simulink model "EffectuatorIntegratedWithDemonstrator"  (R2020a)
settings: Solver=FixedStepDiscrete  StartTime=0.0  StopTime=inf  FixedStep=Ts  RelTol=1e-3
InitFcn:
  | %% Verwende vordefinierte Setpoints (Kreis mit Z-Komponente)
  | 
  | % Config
  | numCircles = 3;
  | scale=6;
  | %Versuch symmetrische Setpunkte zu setzen
  | pointsPerCircle =scale*(4+3*numCircles)+2;
  | 
  | r = 50;
  | m_x = r;
  | m_y = r;
  | 
  | % //
  | s = linspace(0,2*pi,pointsPerCircle);
  | 
  | setPoints_x = [];
  | setPoints_y = [];
  | 
  | for ii=1:numCircles
  | 
  | setPoints_x = [setPoints_x (-cos(s(1:floor(pointsPerCircle / 2))).*r + m_x + 2*r*(ii-1))]; %#ok<AGROW>
  | setPoints_y = [setPoints_y (sin(s).*r+m_y)]; %#ok<AGROW>pointsPerCircle / 2
  | 
  | end
  | 
  | setPoints_x = [setPoints_x flip(setPoints_x(1:end))];
  | 
  | % Loeschen doppelter y-Werte (Kreisuebergang)
  | setPoints_x(pointsPerCircle .* [1:numCircles]) = [];
  | setPoints_y(pointsPerCircle .* [1:numCircles]) = [];
  | 
  | % setPoints_x= [linspace(0,setPoints_x(19),19) setPoints_x(20:end)];
  | % setPoints_y= [linspace(0,setPoints_y(19),19) setPoints_y(20:end)];
  | 
  | % Array Elemente verschieben
  | % setPoints_x = circshift(setPoints_x,-pointsPerCircle/4,2);
  | % setPoints_y = circshift(setPoints_y,-pointsPerCircle/4,2);
  | 
  | z = zeros(1,size(setPoints_x,2));
  | z_x = -5:5;
  | z_y = -z_x.^2 + 25;
  | z_idx = 90;
  | z_idx2 = 210;
  | z(z_idx:z_idx+length(z_x)-1) = z_y;
  | z(z_idx2:z_idx2+length(z_x)-1) = z_y;
  | % z = [z_y z];
  | setPoints_z = z;
  | 
  | % setPoints_x = [zeros(1,length(z_y)) setPoints_x];
  | % setPoints_y = [setPoints_y(1,1)*ones(1,length(z_y)) setPoints_y];
  | 
  | % Umrechnung der Einheiten für Demonstrator
  | % setPoints_x = setPoints_x ./ 1000;
  | % setPoints_y = setPoints_y ./ 1000;
  | % setPoints_z = setPoints_z ./ 1000;
  | 
  | 
  | %{
  | plot(setPoints_x,setPoints_y);
  | fig = figure;
  | ... (+13 lines)
StartFcn:
  | close all;
model workspace (MAT data in the model file):
  MvmtPerfEval_collectVal : Simulink.Parameter (value not decoded)
  MvmtPerfEval_sendOwnVal : Simulink.Parameter (value not decoded)
  PerfEval_numTicks_enable : Simulink.Parameter (value not decoded)
  Segmentregler_I_Gain : Simulink.Parameter (value not decoded)
  Segmentregler_P_Gain : Simulink.Parameter (value not decoded)
  Segmentregler_minVel_enable : Simulink.Parameter (value not decoded)
  Segmentregler_numTicks_enable : Simulink.Parameter (value not decoded)
  Ts : Simulink.Parameter (value not decoded)
  maxPos_x : Simulink.Parameter (value not decoded)
  maxPos_y : Simulink.Parameter (value not decoded)
  maxPos_z : Simulink.Parameter (value not decoded)
  maxVectorLengths : Simulink.Parameter (value not decoded)
  minAllowedVelSaturation : Simulink.Parameter (value not decoded)
  numAxes : Simulink.Parameter (value not decoded)
symbols that are objects in the model workspace (value not decoded): maxPos_x, maxPos_y, maxPos_z, minAllowedVelSaturation, MvmtPerfEval_collectVal, MvmtPerfEval_sendOwnVal, numAxes, PerfEval_numTicks_enable, Segmentregler_I_Gain, Segmentregler_minVel_enable, Segmentregler_numTicks_enable, Segmentregler_P_Gain, Ts
undefined symbols (not defined in the file or in its folder): DiscIntNeverNeededParam, VelOverride
libraries: simulink x20, vrlib x5, sldrtlib x2, xpcrtudplib x2, dspnetwork x2, ptplib x1, etargetslib x1, xpcutilitieslib x1
(part 2 of 5)

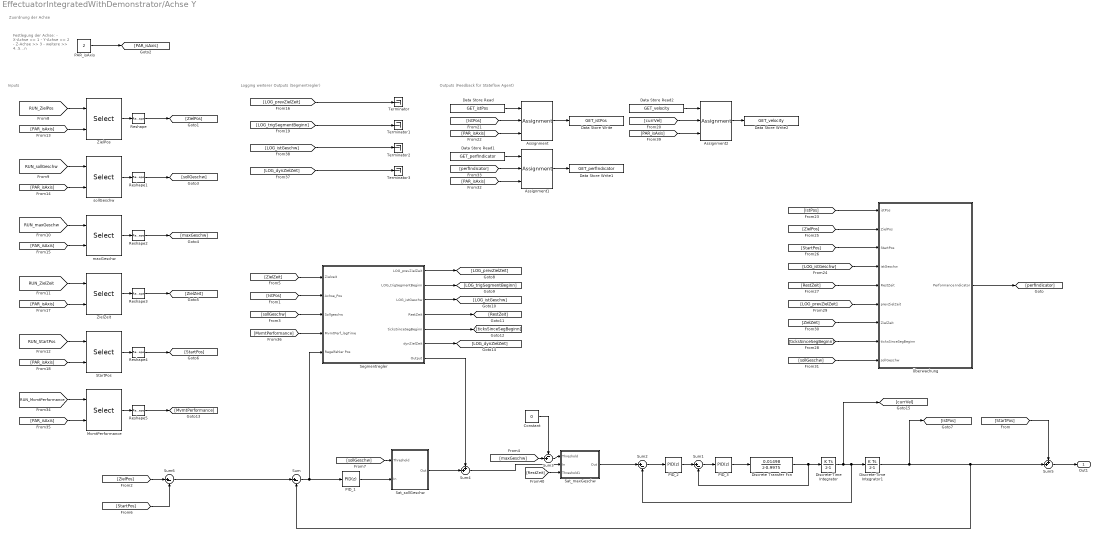
== system EffectuatorIntegratedWithDemonstrator/Achse Y ==
  note: Inputs
  note: Festlegung der Achse:
      | - X-Achse >> 1
      | - Y-Achse >> 2
      | - Z-Achse >> 3
      | - weitere >> 4..5...n
  note: Zuordnung der Achse
  note: Logging weiterer Outputs (Segmentregler)
  note: Outputs (Feedback für Stateflow Agent)
  Assignment : Assignment  DiagnosticForDimensions=Warning  IndexOptions=Index vector (port)  Indices=1  OutputSizes=1
  Assignment1 : Assignment  DiagnosticForDimensions=Warning  IndexOptions=Index vector (port)  Indices=1  OutputSizes=1
  Assignment2 : Assignment  DiagnosticForDimensions=Warning  IndexOptions=Index vector (port)  Indices=1  OutputSizes=1
  Constant : Constant  Value=0
  Data Store Read : DataStoreRead  DataStoreName=GET_istPos
  Data Store Read1 : DataStoreRead  DataStoreName=GET_perfIndicator
  Data Store Read2 : DataStoreRead  DataStoreName=GET_velocity
  Data Store Write : DataStoreWrite  DataStoreName=GET_istPos
  Data Store Write1 : DataStoreWrite  DataStoreName=GET_perfIndicator
  Data Store Write2 : DataStoreWrite  DataStoreName=GET_velocity
  Discrete Transfer Fcn : DiscreteTransferFcn  Numerator=0.01498  Denominator=[1 -0.9975]
  Discrete-Time Integrator : DiscreteIntegrator  SampleTime=-1  ICPrevOutput=DiscIntNeverNeededParam  ICPrevScaledInput=DiscIntNeverNeededParam
  Discrete-Time Integrator1 : DiscreteIntegrator  SampleTime=-1  ICPrevOutput=DiscIntNeverNeededParam  ICPrevScaledInput=DiscIntNeverNeededParam
  MvmtPerformance : Selector  IndexOptions=Index vector (port)  Indices=[1 3]  OutputSizes=1
  PAR_isAxis : Constant  Value=2
  PID_1 : simulink/Continuous/PID Controller  Controller=PID  Form=Parallel  TimeDomain=Discrete-time  UseExternalTs=off  SampleTime=-1  IntegratorMethod=Forward Euler  FilterMethod=Forward Euler  ControllerParametersSource=internal  P=20  I=0  D=0  UseFilter=on  N=100  TunerSelectOption=Transfer Function Based (PID Tuner App)  InitialConditionSource=internal  InitialConditionForIntegrator=0  InitialConditionForFilter=0  DifferentiatorICPrevScaledInput=0  ExternalReset=none  TrackingMode=off  Kt=1  LimitOutput=off  UpperSaturationLimit=inf  LowerSaturationLimit=-inf  LinearizeAsGain=off  AntiWindupMode=none  Kb=1  POutMin=[]  POutMax=[]  IOutMin=[]  IOutMax=[]  DOutMin=[]  DOutMax=[]  NOutMin=[]  NOutMax=[]  SumOutMin=[]  SumOutMax=[]  SaturationOutMin=[]  SaturationOutMax=[]  PParamMin=[]  PParamMax=[]  IParamMin=[]  IParamMax=[]  DParamMin=[]  DParamMax=[]  NParamMin=[]  NParamMax=[]  KbParamMin=[]  KbParamMax=[]  KtParamMin=[]  KtParamMax=[]  KbOutMin=[]  KbOutMax=[]  KtOutMin=[]  KtOutMax=[]  IntegratorOutMin=[]  IntegratorOutMax=[]  FilterOutMin=[]  FilterOutMax=[]  SumI1OutMin=[]  SumI1OutMax=[]  SumI2OutMin=[]  SumI2OutMax=[]  SumI3OutMin=[]  SumI3OutMax=[]  SumI4OutMin=[]  SumI4OutMax=[]  SumDOutMin=[]  SumDOutMax=[]  DifferentiatorOutMin=[]  DifferentiatorOutMax=[]  FilterDiffOutCoefMin=[]  FilterDiffOutCoefMax=[]  ReciprocalOutMin=[]  ReciprocalOutMax=[]  SumDenOutMin=[]  SumDenOutMax=[]  SumNumOutMin=[]  SumNumOutMax=[]  DivideOutMin=[]  DivideOutMax=[]  UdiffTsProdOutMin=[]  UdiffTsProdOutMax=[]  NTsProdOutMin=[]  NTsProdOutMax=[]  UintegralTsProdOutMin=[]  UintegralTsProdOutMax=[]  UngainTsProdOutMin=[]  UngainTsProdOutMax=[]  IntegratorContinuousStateAttributes=''  IntegratorStateMustResolveToSignalObject=off  IntegratorRTWStateStorageClass=Auto  FilterContinuousStateAttributes=''  FilterStateMustResolveToSignalObject=off  FilterRTWStateStorageClass=Auto  ParallelPVariant=InternalParameters  IdealPVariant=Disabled  IVariant=InternalParameters  DVariant=InternalParameters  IntegratorVariant=Discrete  SatVariant=Disabled  AWVariant=Passthrough  PCopyVariant=Disabled  TRVariant=Disabled  FdbkBlocksVariant=Forward  IdealPFdbkVariant=Disabled  SatFdbkVariant=Disabled  DerivativeFilterVariant=ForwardEulerFilter  NVariant=InternalParameters  NCopyVariant=Disabled  FilterICVariant=InternalICsFilter  IntegratorICVariant=InternalICs  ExternalResetVariant=Disabled  TRSumVariant=Passthrough  SumFdbkVariant=Disabled  SumVariant=Sum_PID  TsampFilterVariant=InternalTs  TsampNgainVariant=Passthrough  TsampIntegralVariant=Passthrough
  PID_2 : simulink/Continuous/PID Controller  Controller=PID  Form=Parallel  TimeDomain=Discrete-time  UseExternalTs=off  SampleTime=-1  IntegratorMethod=Forward Euler  FilterMethod=Forward Euler  ControllerParametersSource=internal  P=20  I=1  D=0  UseFilter=on  N=100  TunerSelectOption=Transfer Function Based (PID Tuner App)  InitialConditionSource=internal  InitialConditionForIntegrator=0  InitialConditionForFilter=0  DifferentiatorICPrevScaledInput=0  ExternalReset=none  TrackingMode=off  Kt=1  LimitOutput=off  UpperSaturationLimit=inf  LowerSaturationLimit=-inf  LinearizeAsGain=off  AntiWindupMode=none  Kb=1  POutMin=[]  POutMax=[]  IOutMin=[]  IOutMax=[]  DOutMin=[]  DOutMax=[]  NOutMin=[]  NOutMax=[]  SumOutMin=[]  SumOutMax=[]  SaturationOutMin=[]  SaturationOutMax=[]  PParamMin=[]  PParamMax=[]  IParamMin=[]  IParamMax=[]  DParamMin=[]  DParamMax=[]  NParamMin=[]  NParamMax=[]  KbParamMin=[]  KbParamMax=[]  KtParamMin=[]  KtParamMax=[]  KbOutMin=[]  KbOutMax=[]  KtOutMin=[]  KtOutMax=[]  IntegratorOutMin=[]  IntegratorOutMax=[]  FilterOutMin=[]  FilterOutMax=[]  SumI1OutMin=[]  SumI1OutMax=[]  SumI2OutMin=[]  SumI2OutMax=[]  SumI3OutMin=[]  SumI3OutMax=[]  SumI4OutMin=[]  SumI4OutMax=[]  SumDOutMin=[]  SumDOutMax=[]  DifferentiatorOutMin=[]  DifferentiatorOutMax=[]  FilterDiffOutCoefMin=[]  FilterDiffOutCoefMax=[]  ReciprocalOutMin=[]  ReciprocalOutMax=[]  SumDenOutMin=[]  SumDenOutMax=[]  SumNumOutMin=[]  SumNumOutMax=[]  DivideOutMin=[]  DivideOutMax=[]  UdiffTsProdOutMin=[]  UdiffTsProdOutMax=[]  NTsProdOutMin=[]  NTsProdOutMax=[]  UintegralTsProdOutMin=[]  UintegralTsProdOutMax=[]  UngainTsProdOutMin=[]  UngainTsProdOutMax=[]  IntegratorContinuousStateAttributes=''  IntegratorStateMustResolveToSignalObject=off  IntegratorRTWStateStorageClass=Auto  FilterContinuousStateAttributes=''  FilterStateMustResolveToSignalObject=off  FilterRTWStateStorageClass=Auto  ParallelPVariant=InternalParameters  IdealPVariant=Disabled  IVariant=InternalParameters  DVariant=InternalParameters  IntegratorVariant=Discrete  SatVariant=Disabled  AWVariant=Passthrough  PCopyVariant=Disabled  TRVariant=Disabled  FdbkBlocksVariant=Forward  IdealPFdbkVariant=Disabled  SatFdbkVariant=Disabled  DerivativeFilterVariant=ForwardEulerFilter  NVariant=InternalParameters  NCopyVariant=Disabled  FilterICVariant=InternalICsFilter  IntegratorICVariant=InternalICs  ExternalResetVariant=Disabled  TRSumVariant=Passthrough  SumFdbkVariant=Disabled  SumVariant=Sum_PID  TsampFilterVariant=InternalTs  TsampNgainVariant=Passthrough  TsampIntegralVariant=Passthrough
  PID_3 : simulink/Continuous/PID Controller  Controller=PID  Form=Parallel  TimeDomain=Discrete-time  UseExternalTs=off  SampleTime=-1  IntegratorMethod=Forward Euler  FilterMethod=Forward Euler  ControllerParametersSource=internal  P=20  I=1  D=0  UseFilter=on  N=100  TunerSelectOption=Transfer Function Based (PID Tuner App)  InitialConditionSource=internal  InitialConditionForIntegrator=0  InitialConditionForFilter=0  DifferentiatorICPrevScaledInput=0  ExternalReset=none  TrackingMode=off  Kt=1  LimitOutput=off  UpperSaturationLimit=inf  LowerSaturationLimit=-inf  LinearizeAsGain=off  AntiWindupMode=none  Kb=1  POutMin=[]  POutMax=[]  IOutMin=[]  IOutMax=[]  DOutMin=[]  DOutMax=[]  NOutMin=[]  NOutMax=[]  SumOutMin=[]  SumOutMax=[]  SaturationOutMin=[]  SaturationOutMax=[]  PParamMin=[]  PParamMax=[]  IParamMin=[]  IParamMax=[]  DParamMin=[]  DParamMax=[]  NParamMin=[]  NParamMax=[]  KbParamMin=[]  KbParamMax=[]  KtParamMin=[]  KtParamMax=[]  KbOutMin=[]  KbOutMax=[]  KtOutMin=[]  KtOutMax=[]  IntegratorOutMin=[]  IntegratorOutMax=[]  FilterOutMin=[]  FilterOutMax=[]  SumI1OutMin=[]  SumI1OutMax=[]  SumI2OutMin=[]  SumI2OutMax=[]  SumI3OutMin=[]  SumI3OutMax=[]  SumI4OutMin=[]  SumI4OutMax=[]  SumDOutMin=[]  SumDOutMax=[]  DifferentiatorOutMin=[]  DifferentiatorOutMax=[]  FilterDiffOutCoefMin=[]  FilterDiffOutCoefMax=[]  ReciprocalOutMin=[]  ReciprocalOutMax=[]  SumDenOutMin=[]  SumDenOutMax=[]  SumNumOutMin=[]  SumNumOutMax=[]  DivideOutMin=[]  DivideOutMax=[]  UdiffTsProdOutMin=[]  UdiffTsProdOutMax=[]  NTsProdOutMin=[]  NTsProdOutMax=[]  UintegralTsProdOutMin=[]  UintegralTsProdOutMax=[]  UngainTsProdOutMin=[]  UngainTsProdOutMax=[]  IntegratorContinuousStateAttributes=''  IntegratorStateMustResolveToSignalObject=off  IntegratorRTWStateStorageClass=Auto  FilterContinuousStateAttributes=''  FilterStateMustResolveToSignalObject=off  FilterRTWStateStorageClass=Auto  ParallelPVariant=InternalParameters  IdealPVariant=Disabled  IVariant=InternalParameters  DVariant=InternalParameters  IntegratorVariant=Discrete  SatVariant=Disabled  AWVariant=Passthrough  PCopyVariant=Disabled  TRVariant=Disabled  FdbkBlocksVariant=Forward  IdealPFdbkVariant=Disabled  SatFdbkVariant=Disabled  DerivativeFilterVariant=ForwardEulerFilter  NVariant=InternalParameters  NCopyVariant=Disabled  FilterICVariant=InternalICsFilter  IntegratorICVariant=InternalICs  ExternalResetVariant=Disabled  TRSumVariant=Passthrough  SumFdbkVariant=Disabled  SumVariant=Sum_PID  TsampFilterVariant=InternalTs  TsampNgainVariant=Passthrough  TsampIntegralVariant=Passthrough
  Reshape{,1..5} (6 alike) : Reshape
  Sat_maxGeschw : Subsystem
  Sat_sollGeschw : Subsystem
  Segmentregler : Subsystem
  StartPos : Selector  IndexOptions=Index vector (port)  Indices=[1 3]  OutputSizes=1
  Sum{,1..2,6} (4 alike) : Sum  Inputs=|+-
  Sum3 : Sum  Inputs=-+|
  Sum4 : Sum  Inputs=++|
  Sum5 : Sum  Inputs=++|
  Terminator{,1..3} (4 alike) : Terminator
  ZielPos : Selector  IndexOptions=Index vector (port)  Indices=[1 3]  OutputSizes=1
  ZielZeit : Selector  IndexOptions=Index vector (port)  Indices=[1 3]  OutputSizes=1
  maxGeschw : Selector  IndexOptions=Index vector (port)  Indices=[1 3]  OutputSizes=1
  sollGeschw : Selector  IndexOptions=Index vector (port)  Indices=[1 3]  OutputSizes=1
  Überwachung : Subsystem
  Out1 : Outport  VectorParamsAs1DForOutWhenUnconnected=off
  wires:
  [LOG_dynZielZeit] -> Terminator3/1
  Segmentregler/6(dynZielZeit) -> [LOG_dynZielZeit]
  [MvmtPerformance] -> Segmentregler/4(MvmtPerf_lagTime)
  [PAR_isAxis] -> MvmtPerformance/2
  [RUN_MvmtPerformance] -> MvmtPerformance/1
  MvmtPerformance/1 -> Reshape5/1
  Reshape5/1 -> [MvmtPerformance]
  [sollGeschw] -> Überwachung/9(sollGeschw)
  [ticksSinceSegBeginn] -> Überwachung/8(ticksSinceSegBeginn)
  Segmentregler/5(ticksSinceSegBeginn) -> [ticksSinceSegBeginn]
  Überwachung/1(Performance Indicator) -> [perfIndicator]
  Data Store Read1/1 -> Assignment1/1
  [perfIndicator] -> Assignment1/2
  [PAR_isAxis] -> Assignment1/3
  Assignment1/1 -> Data Store Write1/1
  [ZielZeit] -> Überwachung/7(ZielZeit)
  [LOG_prevZielZeit] -> Überwachung/6(prevZielZeit)
  [RestZeit] -> Überwachung/5(RestZeit)
  [LOG_istGeschw] -> Überwachung/4(istGeschw)
  [StartPos] -> Überwachung/3(StartPos)
  [ZielPos] -> Überwachung/2(ZielPos)
  [IstPos] -> Überwachung/1(istPos)
  Constant/1 -> Sum3/1
  Sum3/1 -> Sat_maxGeschw/1(Threshold)
  [maxGeschw] -> Sum3/2
  Segmentregler/4(RestZeit) -> [RestZeit]
  Assignment/1 -> Data Store Write/1
  [PAR_isAxis] -> Assignment/3
  [IstPos] -> Assignment/2
  Data Store Read/1 -> Assignment/1
  Reshape3/1 -> [ZielZeit]
  Reshape4/1 -> [StartPos]
  Reshape2/1 -> [maxGeschw]
  Reshape1/1 -> [sollGeschw]
  Reshape/1 -> [ZielPos]
  [LOG_trigSegmentBeginn] -> Terminator1/1
  [LOG_prevZielZeit] -> Terminator/1
  Segmentregler/3(LOG_istGeschw) -> [LOG_istGeschw]
  Segmentregler/2(LOG_trigSegmentBeginn) -> [LOG_trigSegmentBeginn]
  Segmentregler/1(LOG_prevZielZeit) -> [LOG_prevZielZeit]
  StartPos/1 -> Reshape4/1
  [RUN_StartPos] -> StartPos/1
  [PAR_isAxis] -> StartPos/2
  [PAR_isAxis] -> ZielZeit/2
  [RUN_ZielZeit] -> ZielZeit/1
  ZielZeit/1 -> Reshape3/1
  maxGeschw/1 -> Reshape2/1
  [RUN_maxGeschw] -> maxGeschw/1
  [PAR_isAxis] -> maxGeschw/2
  [PAR_isAxis] -> sollGeschw/2
  [RUN_sollGeschw] -> sollGeschw/1
  sollGeschw/1 -> Reshape1/1
  ZielPos/1 -> Reshape/1
  [RUN_ZielPos] -> ZielPos/1
  [PAR_isAxis] -> ZielPos/2
  PAR_isAxis/1 -> [PAR_isAxis]
  [sollGeschw] -> Sat_sollGeschw/1(Threshold)
  [sollGeschw] -> Segmentregler/3(Sollgeschw)
  [StartPos] -> Sum6/2
  [StartPos] -> Sum5/1
  Segmentregler/7(Output) -> Sum4/1
  [IstPos] -> Segmentregler/2(Achse_Pos)
  [ZielZeit] -> Segmentregler/1(Zielzeit)
  [ZielPos] -> Sum6/1
  Sum5/1 -> Out1/1
  Discrete-Time Integrator1/1 -> Sum/2, Sum5/2, [IstPos]
  Sat_maxGeschw/1(Out) -> Sum2/1
  PID_2/1 -> Sum1/1
  Sum1/1 -> PID_3/1
  Discrete-Time Integrator/1 -> [currVel], Sum2/2, Discrete-Time Integrator1/1
  Sum6/1 -> Sum/1
  Sum2/1 -> PID_2/1
  Discrete Transfer Fcn/1 -> Sum1/2, Discrete-Time Integrator/1
  PID_3/1 -> Discrete Transfer Fcn/1
  Sum4/1 -> Sat_maxGeschw/2(In)
  Sat_sollGeschw/1(Out) -> Sum4/2
  PID_1/1 -> Sat_sollGeschw/2(In)
  Sum/1 -> PID_1/1, Segmentregler/5(Regelfehler Pos)
  [LOG_istGeschw] -> Terminator2/1
  Assignment2/1 -> Data Store Write2/1
  Data Store Read2/1 -> Assignment2/1
  [PAR_isAxis] -> Assignment2/3
  [currVel] -> Assignment2/2
  [RestZeit] -> Sat_maxGeschw/3(Threshold1)

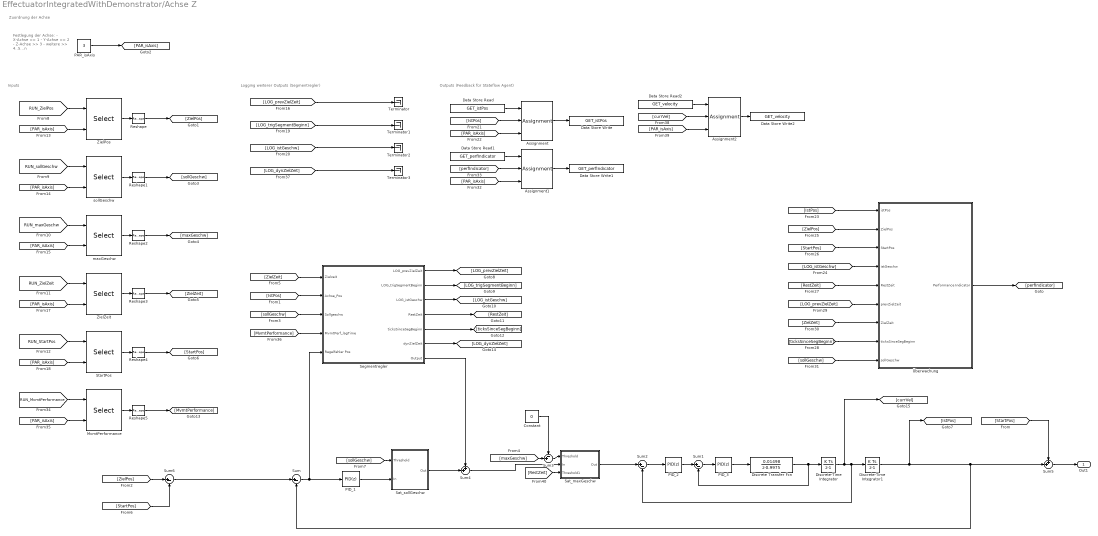
== system EffectuatorIntegratedWithDemonstrator/Achse Z ==
  note: Outputs (Feedback für Stateflow Agent)
  note: Logging weiterer Outputs (Segmentregler)
  note: Zuordnung der Achse
  note: Festlegung der Achse:
      | - X-Achse >> 1
      | - Y-Achse >> 2
      | - Z-Achse >> 3
      | - weitere >> 4..5...n
  note: Inputs
  Assignment : Assignment  DiagnosticForDimensions=Warning  IndexOptions=Index vector (port)  Indices=1  OutputSizes=1
  Assignment1 : Assignment  DiagnosticForDimensions=Warning  IndexOptions=Index vector (port)  Indices=1  OutputSizes=1
  Assignment2 : Assignment  DiagnosticForDimensions=Warning  IndexOptions=Index vector (port)  Indices=1  OutputSizes=1
  Constant : Constant  Value=0
  Data Store Read : DataStoreRead  DataStoreName=GET_istPos
  Data Store Read1 : DataStoreRead  DataStoreName=GET_perfIndicator
  Data Store Read2 : DataStoreRead  DataStoreName=GET_velocity
  Data Store Write : DataStoreWrite  DataStoreName=GET_istPos
  Data Store Write1 : DataStoreWrite  DataStoreName=GET_perfIndicator
  Data Store Write2 : DataStoreWrite  DataStoreName=GET_velocity
  Discrete Transfer Fcn : DiscreteTransferFcn  Numerator=0.01498  Denominator=[1 -0.9975]
  Discrete-Time Integrator : DiscreteIntegrator  SampleTime=-1  ICPrevOutput=DiscIntNeverNeededParam  ICPrevScaledInput=DiscIntNeverNeededParam
  Discrete-Time Integrator1 : DiscreteIntegrator  SampleTime=-1  ICPrevOutput=DiscIntNeverNeededParam  ICPrevScaledInput=DiscIntNeverNeededParam
  MvmtPerformance : Selector  IndexOptions=Index vector (port)  Indices=[1 3]  OutputSizes=1
  PAR_isAxis : Constant  Value=3
  PID_1 : simulink/Continuous/PID Controller  Controller=PID  Form=Parallel  TimeDomain=Discrete-time  UseExternalTs=off  SampleTime=-1  IntegratorMethod=Forward Euler  FilterMethod=Forward Euler  ControllerParametersSource=internal  P=20  I=0  D=0  UseFilter=on  N=100  TunerSelectOption=Transfer Function Based (PID Tuner App)  InitialConditionSource=internal  InitialConditionForIntegrator=0  InitialConditionForFilter=0  DifferentiatorICPrevScaledInput=0  ExternalReset=none  TrackingMode=off  Kt=1  LimitOutput=off  UpperSaturationLimit=inf  LowerSaturationLimit=-inf  LinearizeAsGain=off  AntiWindupMode=none  Kb=1  POutMin=[]  POutMax=[]  IOutMin=[]  IOutMax=[]  DOutMin=[]  DOutMax=[]  NOutMin=[]  NOutMax=[]  SumOutMin=[]  SumOutMax=[]  SaturationOutMin=[]  SaturationOutMax=[]  PParamMin=[]  PParamMax=[]  IParamMin=[]  IParamMax=[]  DParamMin=[]  DParamMax=[]  NParamMin=[]  NParamMax=[]  KbParamMin=[]  KbParamMax=[]  KtParamMin=[]  KtParamMax=[]  KbOutMin=[]  KbOutMax=[]  KtOutMin=[]  KtOutMax=[]  IntegratorOutMin=[]  IntegratorOutMax=[]  FilterOutMin=[]  FilterOutMax=[]  SumI1OutMin=[]  SumI1OutMax=[]  SumI2OutMin=[]  SumI2OutMax=[]  SumI3OutMin=[]  SumI3OutMax=[]  SumI4OutMin=[]  SumI4OutMax=[]  SumDOutMin=[]  SumDOutMax=[]  DifferentiatorOutMin=[]  DifferentiatorOutMax=[]  FilterDiffOutCoefMin=[]  FilterDiffOutCoefMax=[]  ReciprocalOutMin=[]  ReciprocalOutMax=[]  SumDenOutMin=[]  SumDenOutMax=[]  SumNumOutMin=[]  SumNumOutMax=[]  DivideOutMin=[]  DivideOutMax=[]  UdiffTsProdOutMin=[]  UdiffTsProdOutMax=[]  NTsProdOutMin=[]  NTsProdOutMax=[]  UintegralTsProdOutMin=[]  UintegralTsProdOutMax=[]  UngainTsProdOutMin=[]  UngainTsProdOutMax=[]  IntegratorContinuousStateAttributes=''  IntegratorStateMustResolveToSignalObject=off  IntegratorRTWStateStorageClass=Auto  FilterContinuousStateAttributes=''  FilterStateMustResolveToSignalObject=off  FilterRTWStateStorageClass=Auto  ParallelPVariant=InternalParameters  IdealPVariant=Disabled  IVariant=InternalParameters  DVariant=InternalParameters  IntegratorVariant=Discrete  SatVariant=Disabled  AWVariant=Passthrough  PCopyVariant=Disabled  TRVariant=Disabled  FdbkBlocksVariant=Forward  IdealPFdbkVariant=Disabled  SatFdbkVariant=Disabled  DerivativeFilterVariant=ForwardEulerFilter  NVariant=InternalParameters  NCopyVariant=Disabled  FilterICVariant=InternalICsFilter  IntegratorICVariant=InternalICs  ExternalResetVariant=Disabled  TRSumVariant=Passthrough  SumFdbkVariant=Disabled  SumVariant=Sum_PID  TsampFilterVariant=InternalTs  TsampNgainVariant=Passthrough  TsampIntegralVariant=Passthrough
  PID_2 : simulink/Continuous/PID Controller  Controller=PID  Form=Parallel  TimeDomain=Discrete-time  UseExternalTs=off  SampleTime=-1  IntegratorMethod=Forward Euler  FilterMethod=Forward Euler  ControllerParametersSource=internal  P=20  I=1  D=0  UseFilter=on  N=100  TunerSelectOption=Transfer Function Based (PID Tuner App)  InitialConditionSource=internal  InitialConditionForIntegrator=0  InitialConditionForFilter=0  DifferentiatorICPrevScaledInput=0  ExternalReset=none  TrackingMode=off  Kt=1  LimitOutput=off  UpperSaturationLimit=inf  LowerSaturationLimit=-inf  LinearizeAsGain=off  AntiWindupMode=none  Kb=1  POutMin=[]  POutMax=[]  IOutMin=[]  IOutMax=[]  DOutMin=[]  DOutMax=[]  NOutMin=[]  NOutMax=[]  SumOutMin=[]  SumOutMax=[]  SaturationOutMin=[]  SaturationOutMax=[]  PParamMin=[]  PParamMax=[]  IParamMin=[]  IParamMax=[]  DParamMin=[]  DParamMax=[]  NParamMin=[]  NParamMax=[]  KbParamMin=[]  KbParamMax=[]  KtParamMin=[]  KtParamMax=[]  KbOutMin=[]  KbOutMax=[]  KtOutMin=[]  KtOutMax=[]  IntegratorOutMin=[]  IntegratorOutMax=[]  FilterOutMin=[]  FilterOutMax=[]  SumI1OutMin=[]  SumI1OutMax=[]  SumI2OutMin=[]  SumI2OutMax=[]  SumI3OutMin=[]  SumI3OutMax=[]  SumI4OutMin=[]  SumI4OutMax=[]  SumDOutMin=[]  SumDOutMax=[]  DifferentiatorOutMin=[]  DifferentiatorOutMax=[]  FilterDiffOutCoefMin=[]  FilterDiffOutCoefMax=[]  ReciprocalOutMin=[]  ReciprocalOutMax=[]  SumDenOutMin=[]  SumDenOutMax=[]  SumNumOutMin=[]  SumNumOutMax=[]  DivideOutMin=[]  DivideOutMax=[]  UdiffTsProdOutMin=[]  UdiffTsProdOutMax=[]  NTsProdOutMin=[]  NTsProdOutMax=[]  UintegralTsProdOutMin=[]  UintegralTsProdOutMax=[]  UngainTsProdOutMin=[]  UngainTsProdOutMax=[]  IntegratorContinuousStateAttributes=''  IntegratorStateMustResolveToSignalObject=off  IntegratorRTWStateStorageClass=Auto  FilterContinuousStateAttributes=''  FilterStateMustResolveToSignalObject=off  FilterRTWStateStorageClass=Auto  ParallelPVariant=InternalParameters  IdealPVariant=Disabled  IVariant=InternalParameters  DVariant=InternalParameters  IntegratorVariant=Discrete  SatVariant=Disabled  AWVariant=Passthrough  PCopyVariant=Disabled  TRVariant=Disabled  FdbkBlocksVariant=Forward  IdealPFdbkVariant=Disabled  SatFdbkVariant=Disabled  DerivativeFilterVariant=ForwardEulerFilter  NVariant=InternalParameters  NCopyVariant=Disabled  FilterICVariant=InternalICsFilter  IntegratorICVariant=InternalICs  ExternalResetVariant=Disabled  TRSumVariant=Passthrough  SumFdbkVariant=Disabled  SumVariant=Sum_PID  TsampFilterVariant=InternalTs  TsampNgainVariant=Passthrough  TsampIntegralVariant=Passthrough
  PID_3 : simulink/Continuous/PID Controller  Controller=PID  Form=Parallel  TimeDomain=Discrete-time  UseExternalTs=off  SampleTime=-1  IntegratorMethod=Forward Euler  FilterMethod=Forward Euler  ControllerParametersSource=internal  P=20  I=1  D=0  UseFilter=on  N=100  TunerSelectOption=Transfer Function Based (PID Tuner App)  InitialConditionSource=internal  InitialConditionForIntegrator=0  InitialConditionForFilter=0  DifferentiatorICPrevScaledInput=0  ExternalReset=none  TrackingMode=off  Kt=1  LimitOutput=off  UpperSaturationLimit=inf  LowerSaturationLimit=-inf  LinearizeAsGain=off  AntiWindupMode=none  Kb=1  POutMin=[]  POutMax=[]  IOutMin=[]  IOutMax=[]  DOutMin=[]  DOutMax=[]  NOutMin=[]  NOutMax=[]  SumOutMin=[]  SumOutMax=[]  SaturationOutMin=[]  SaturationOutMax=[]  PParamMin=[]  PParamMax=[]  IParamMin=[]  IParamMax=[]  DParamMin=[]  DParamMax=[]  NParamMin=[]  NParamMax=[]  KbParamMin=[]  KbParamMax=[]  KtParamMin=[]  KtParamMax=[]  KbOutMin=[]  KbOutMax=[]  KtOutMin=[]  KtOutMax=[]  IntegratorOutMin=[]  IntegratorOutMax=[]  FilterOutMin=[]  FilterOutMax=[]  SumI1OutMin=[]  SumI1OutMax=[]  SumI2OutMin=[]  SumI2OutMax=[]  SumI3OutMin=[]  SumI3OutMax=[]  SumI4OutMin=[]  SumI4OutMax=[]  SumDOutMin=[]  SumDOutMax=[]  DifferentiatorOutMin=[]  DifferentiatorOutMax=[]  FilterDiffOutCoefMin=[]  FilterDiffOutCoefMax=[]  ReciprocalOutMin=[]  ReciprocalOutMax=[]  SumDenOutMin=[]  SumDenOutMax=[]  SumNumOutMin=[]  SumNumOutMax=[]  DivideOutMin=[]  DivideOutMax=[]  UdiffTsProdOutMin=[]  UdiffTsProdOutMax=[]  NTsProdOutMin=[]  NTsProdOutMax=[]  UintegralTsProdOutMin=[]  UintegralTsProdOutMax=[]  UngainTsProdOutMin=[]  UngainTsProdOutMax=[]  IntegratorContinuousStateAttributes=''  IntegratorStateMustResolveToSignalObject=off  IntegratorRTWStateStorageClass=Auto  FilterContinuousStateAttributes=''  FilterStateMustResolveToSignalObject=off  FilterRTWStateStorageClass=Auto  ParallelPVariant=InternalParameters  IdealPVariant=Disabled  IVariant=InternalParameters  DVariant=InternalParameters  IntegratorVariant=Discrete  SatVariant=Disabled  AWVariant=Passthrough  PCopyVariant=Disabled  TRVariant=Disabled  FdbkBlocksVariant=Forward  IdealPFdbkVariant=Disabled  SatFdbkVariant=Disabled  DerivativeFilterVariant=ForwardEulerFilter  NVariant=InternalParameters  NCopyVariant=Disabled  FilterICVariant=InternalICsFilter  IntegratorICVariant=InternalICs  ExternalResetVariant=Disabled  TRSumVariant=Passthrough  SumFdbkVariant=Disabled  SumVariant=Sum_PID  TsampFilterVariant=InternalTs  TsampNgainVariant=Passthrough  TsampIntegralVariant=Passthrough
  Reshape{,1..5} (6 alike) : Reshape
  Sat_maxGeschw : Subsystem
  Sat_sollGeschw : Subsystem
  Segmentregler : Subsystem
  StartPos : Selector  IndexOptions=Index vector (port)  Indices=[1 3]  OutputSizes=1
  Sum{,1..2,6} (4 alike) : Sum  Inputs=|+-
  Sum3 : Sum  Inputs=-+|
  Sum4 : Sum  Inputs=++|
  Sum5 : Sum  Inputs=++|
  Terminator{,1..3} (4 alike) : Terminator
  ZielPos : Selector  IndexOptions=Index vector (port)  Indices=[1 3]  OutputSizes=1
  ZielZeit : Selector  IndexOptions=Index vector (port)  Indices=[1 3]  OutputSizes=1
  maxGeschw : Selector  IndexOptions=Index vector (port)  Indices=[1 3]  OutputSizes=1
  sollGeschw : Selector  IndexOptions=Index vector (port)  Indices=[1 3]  OutputSizes=1
  Überwachung : Subsystem
  Out1 : Outport  VectorParamsAs1DForOutWhenUnconnected=off
  wires:
  Sum/1 -> Segmentregler/5(Regelfehler Pos), PID_1/1
  PID_1/1 -> Sat_sollGeschw/2(In)
  Sat_sollGeschw/1(Out) -> Sum4/2
  Sum4/1 -> Sat_maxGeschw/2(In)
  PID_3/1 -> Discrete Transfer Fcn/1
  Discrete Transfer Fcn/1 -> Discrete-Time Integrator/1, Sum1/2
  Sum2/1 -> PID_2/1
  Sum6/1 -> Sum/1
  Discrete-Time Integrator/1 -> [currVel], Discrete-Time Integrator1/1, Sum2/2
  Sum1/1 -> PID_3/1
  PID_2/1 -> Sum1/1
  Discrete-Time Integrator1/1 -> [IstPos], Sum5/2, Sum/2
  Sum5/1 -> Out1/1
  [ZielPos] -> Sum6/1
  [ZielZeit] -> Segmentregler/1(Zielzeit)
  [IstPos] -> Segmentregler/2(Achse_Pos)
  Segmentregler/7(Output) -> Sum4/1
  [StartPos] -> Sum5/1
  [StartPos] -> Sum6/2
  [sollGeschw] -> Segmentregler/3(Sollgeschw)
  [sollGeschw] -> Sat_sollGeschw/1(Threshold)
  PAR_isAxis/1 -> [PAR_isAxis]
  [PAR_isAxis] -> ZielPos/2
  [RUN_ZielPos] -> ZielPos/1
  ZielPos/1 -> Reshape/1
  sollGeschw/1 -> Reshape1/1
  [RUN_sollGeschw] -> sollGeschw/1
  [PAR_isAxis] -> sollGeschw/2
  [PAR_isAxis] -> maxGeschw/2
  [RUN_maxGeschw] -> maxGeschw/1
  maxGeschw/1 -> Reshape2/1
  ZielZeit/1 -> Reshape3/1
  [RUN_ZielZeit] -> ZielZeit/1
  [PAR_isAxis] -> ZielZeit/2
  [PAR_isAxis] -> StartPos/2
  [RUN_StartPos] -> StartPos/1
  StartPos/1 -> Reshape4/1
  Segmentregler/1(LOG_prevZielZeit) -> [LOG_prevZielZeit]
  Segmentregler/2(LOG_trigSegmentBeginn) -> [LOG_trigSegmentBeginn]
  Segmentregler/3(LOG_istGeschw) -> [LOG_istGeschw]
  [LOG_prevZielZeit] -> Terminator/1
  [LOG_trigSegmentBeginn] -> Terminator1/1
  Reshape/1 -> [ZielPos]
  Reshape1/1 -> [sollGeschw]
  Reshape2/1 -> [maxGeschw]
  Reshape4/1 -> [StartPos]
  Reshape3/1 -> [ZielZeit]
  Data Store Read/1 -> Assignment/1
  [IstPos] -> Assignment/2
  [PAR_isAxis] -> Assignment/3
  Assignment/1 -> Data Store Write/1
  Segmentregler/4(RestZeit) -> [RestZeit]
  [maxGeschw] -> Sum3/2
  Sum3/1 -> Sat_maxGeschw/1(Threshold)
  Constant/1 -> Sum3/1
  [IstPos] -> Überwachung/1(istPos)
  [ZielPos] -> Überwachung/2(ZielPos)
  [StartPos] -> Überwachung/3(StartPos)
  [LOG_istGeschw] -> Überwachung/4(istGeschw)
  [RestZeit] -> Überwachung/5(RestZeit)
  [LOG_prevZielZeit] -> Überwachung/6(prevZielZeit)
  [ZielZeit] -> Überwachung/7(ZielZeit)
  Assignment1/1 -> Data Store Write1/1
  [PAR_isAxis] -> Assignment1/3
  [perfIndicator] -> Assignment1/2
  Data Store Read1/1 -> Assignment1/1
  Überwachung/1(Performance Indicator) -> [perfIndicator]
  Segmentregler/5(ticksSinceSegBeginn) -> [ticksSinceSegBeginn]
  [ticksSinceSegBeginn] -> Überwachung/8(ticksSinceSegBeginn)
  [sollGeschw] -> Überwachung/9(sollGeschw)
  Reshape5/1 -> [MvmtPerformance]
  MvmtPerformance/1 -> Reshape5/1
  [RUN_MvmtPerformance] -> MvmtPerformance/1
  [PAR_isAxis] -> MvmtPerformance/2
  [MvmtPerformance] -> Segmentregler/4(MvmtPerf_lagTime)
  Segmentregler/6(dynZielZeit) -> [LOG_dynZielZeit]
  [LOG_dynZielZeit] -> Terminator3/1
  [LOG_istGeschw] -> Terminator2/1
  Assignment2/1 -> Data Store Write2/1
  Data Store Read2/1 -> Assignment2/1
  [PAR_isAxis] -> Assignment2/3
  [currVel] -> Assignment2/2
  [RestZeit] -> Sat_maxGeschw/3(Threshold1)
  Sat_maxGeschw/1(Out) -> Sum2/1
